simulink model "framework_sim"  (R2019b)
settings: Solver=FixedStepDiscrete  StartTime=T0  StopTime=Tf  FixedStep=Ts  EnableMultiTasking=on
model workspace (MAT data in the model file):
  aKalman : Simulink.Parameter (value not decoded)
  slipEnabler : Simulink.Parameter (value not decoded)
values from neighbouring files (symbols this model uses):
  enable_onlinePlots = 0    [main_framework.m]
  enable_zoom = 0    [main_framework.m]
  HLP_sampleTime = planner.replan_time    [main_framework.m]
  Kb = 10    [main_framework.m]
  Kd_vals = PID_Gain_Scheduling(:,4)    [main_framework.m]
  Ki_vals = PID_Gain_Scheduling(:,3)    [main_framework.m]
  Kp_vals = PID_Gain_Scheduling(:,2)    [main_framework.m]
  latContr_select = 4    [select_lateralController.m]
  mapObjects = scenario.scenario_data.mapObjects    [main_framework.m]
  N_vals = PID_Gain_Scheduling(:,5)    [main_framework.m]
  refRoute_fewPoints = referencePath_fewPoints.refRoute_fewPoints    [main_framework.m]    (also in refPath_poses_fewPoints.mat = [5 34.9682620653 63.3276365473 92.153562059 121.414282249 15; routePlanner.m = [x_cloth_refPath_fewPoints',y_cloth_refPath_fewPoints',theta)
  speed_vals_PID_sched = PID_Gain_Scheduling(:,1)    [main_framework.m]
  tau_D = vehicle_data.steering_system.tau_D    [dataAnalysis.m]    (also in main_framework.m)
  Ts = simulationPars.times.step_size    [main_framework.m]
  vehicle_data = getVehicleDataStruct()    [aeroModel.m]    (also in loadInitialConditions.m; longitSlipModel.m; main_framework.m; perfectAcker.m)
  X0 = loadInitialConditions    [main_framework.m]
undefined symbols (not defined in the file or in its folder): DiscIntNeverNeededParam, loadInitialPose
libraries: simulink_extras x16, drivingvehiclecontroller x2, simulink x1
(part 3 of 3)

== matlab function framework_sim/Lateral Controller/Arc Path Following Controller/Arc Path Following Controller ==
  data: target_Point input; delta output; pose input; endOfCircuit input
function delta  = arcPathFollowController(target_Point,pose,endOfCircuit)

    coder.extrinsic('round');

    % Load vehicle params
    vehicle_params = getVehicleDataStruct();
    Lf = vehicle_params.vehicle.Lf;        
    Lr = vehicle_params.vehicle.Lr;    
    L  = Lf + Lr;  % [m] vehicle wheelbase
    
    % Current vehicle center of mass pose 
    x_C     = pose(1);
    y_C     = pose(2);
    theta_C = pose(3);  % vehicle attitude (in radians)
     
    % Rotation matrix from vehicle frame to absolute frame
    Rot_mat = [cos(theta_C), -sin(theta_C); ...
               sin(theta_C),  cos(theta_C)];
    
    % Point of the vehicle in correspondence with the rear axle
    x_R = x_C - Lr*cos(theta_C);
    y_R = y_C - Lr*sin(theta_C);
    current_point = [x_R y_R];
    
    % Express the current_point in the vehicle frame
    current_point_vehFrame = [-Lr,0];
    
    % Distance from the current position to the target point
    distFromTarget = sqrt((target_Point(1)-current_point(1))^2 + (target_Point(2)-current_point(2))^2);
    
    % Express the target_Point in the vehicle frame
    target_Point_vehFrame = Rot_mat'*(target_Point(1:2)' - current_point');
    
    % Angle measured w.r.t. the vehicle reference frame
    gamma = atan2((target_Point_vehFrame(2)-current_point_vehFrame(2))/distFromTarget,(target_Point_vehFrame(1)-current_point_vehFrame(1))/distFromTarget);
    
    % Required curvature radius
    R = 0.5*distFromTarget/sin(gamma);
   
    if (~endOfCircuit)
        delta = atan(L/R);    
    else
        delta = 0;
    end

end
